simulink model "Dnote3lv3rd"  (R2016b)
settings: Solver=FixedStepDiscrete  StartTime=0.0  StopTime=simtime  RelTol=1e-3  EnableMultiTasking=on
PreLoadFcn:
  | simtime=0.0034;
undefined symbols (not defined in the file): Amp, fdesignblkfcn, Fin, Fs, FSC, gcbh, N, p, sw1, Ts
libraries: simulink x153, dspsnks4 x2, dspfdesign x1, dspvision x1, dsparch4 x1, dspmlti4 x1
(part 2 of 3)

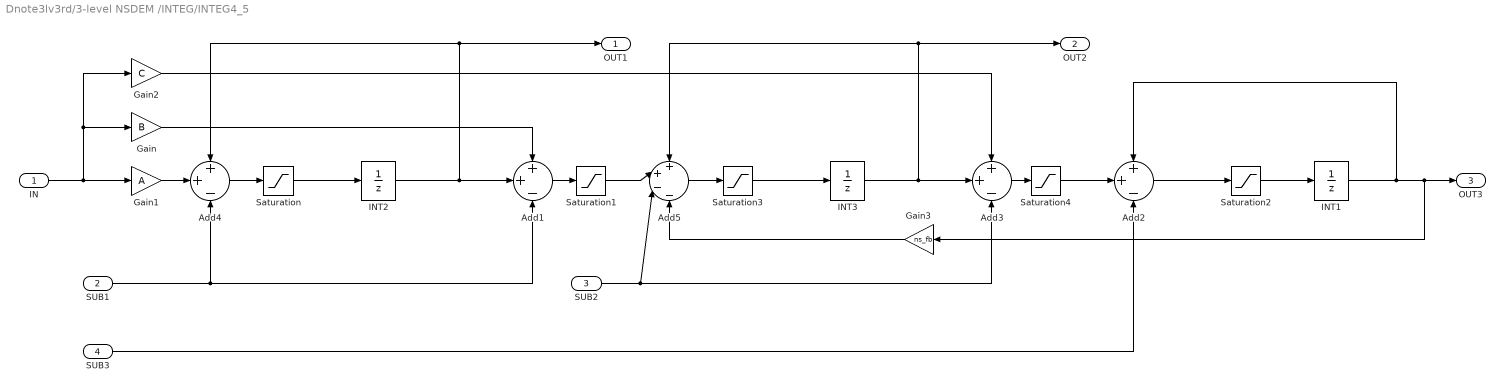
== system Dnote3lv3rd/3-level NSDEM /INTEG/INTEG4_5 ==
  IN : Inport
  SUB1 : Inport  Port=2
  SUB2 : Inport  Port=3
  SUB3 : Inport  Port=4
  Add{1..4} (4 alike) : Sum  Inputs=++-
  Add5 : Sum  Inputs=++--
  Gain : Gain  Gain=B
  Gain1 : Gain  Gain=A
  Gain2 : Gain  Gain=C
  Gain3 : Gain  Gain=ns_fb
  INT1 : UnitDelay  SampleTime=Ts
  INT2 : UnitDelay  SampleTime=Ts
  INT3 : UnitDelay  SampleTime=Ts
  Saturation{,1..4} (5 alike) : Saturate  UpperLimit=SAT  LowerLimit=-SAT
  OUT1 : Outport
  OUT2 : Outport  Port=2
  OUT3 : Outport  Port=3
  wires:
  Gain1/1 -> Add4/2
  Saturation1/1 -> Add5/2
  Saturation4/1 -> Add2/2
  Gain2/1 -> Add3/1
  Add3/1 -> Saturation4/1
  SUB2/1 -> Add3/3, Add5/3
  Add5/1 -> Saturation3/1
  Add2/1 -> Saturation2/1
  Gain/1 -> Add1/1
  Add1/1 -> Saturation1/1
  IN/1 -> Gain1/1, Gain2/1, Gain/1
  SUB1/1 -> Add4/3, Add1/3
  Add4/1 -> Saturation/1
  SUB3/1 -> Add2/3
  Gain3/1 -> Add5/4
  INT1/1 -> Add2/1, Gain3/1, OUT3/1
  INT3/1 -> Add3/2, OUT2/1, Add5/1
  Saturation2/1 -> INT1/1
  INT2/1 -> OUT1/1, Add4/1, Add1/2
  Saturation/1 -> INT2/1
  Saturation3/1 -> INT3/1

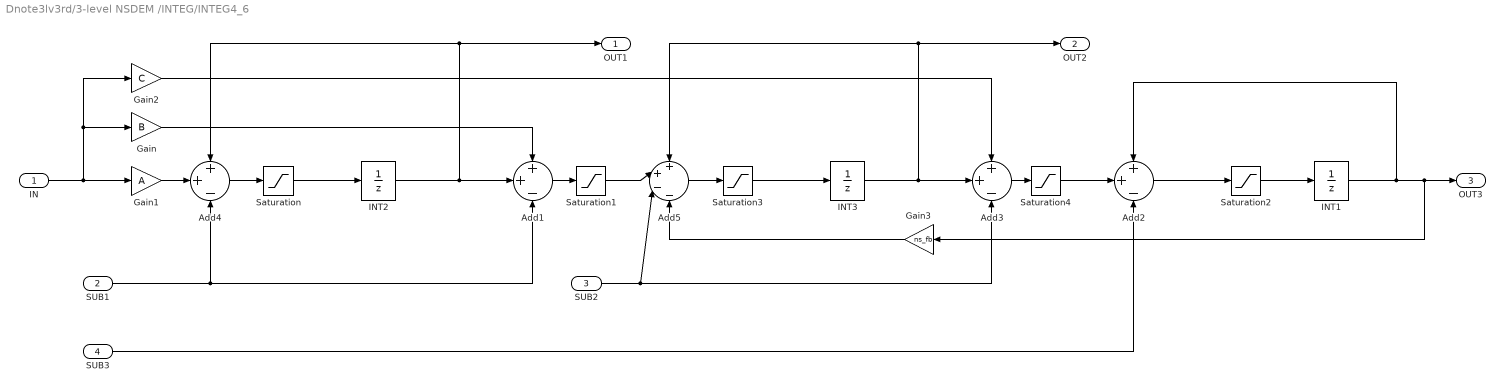
== system Dnote3lv3rd/3-level NSDEM /INTEG/INTEG4_6 ==
  IN : Inport
  SUB1 : Inport  Port=2
  SUB2 : Inport  Port=3
  SUB3 : Inport  Port=4
  Add{1..4} (4 alike) : Sum  Inputs=++-
  Add5 : Sum  Inputs=++--
  Gain : Gain  Gain=B
  Gain1 : Gain  Gain=A
  Gain2 : Gain  Gain=C
  Gain3 : Gain  Gain=ns_fb
  INT1 : UnitDelay  SampleTime=Ts
  INT2 : UnitDelay  SampleTime=Ts
  INT3 : UnitDelay  SampleTime=Ts
  Saturation{,1..4} (5 alike) : Saturate  UpperLimit=SAT  LowerLimit=-SAT
  OUT1 : Outport
  OUT2 : Outport  Port=2
  OUT3 : Outport  Port=3
  wires:
  Gain1/1 -> Add4/2
  Saturation1/1 -> Add5/2
  Saturation4/1 -> Add2/2
  Gain2/1 -> Add3/1
  Add3/1 -> Saturation4/1
  SUB2/1 -> Add3/3, Add5/3
  Add5/1 -> Saturation3/1
  Add2/1 -> Saturation2/1
  Gain/1 -> Add1/1
  Add1/1 -> Saturation1/1
  IN/1 -> Gain1/1, Gain2/1, Gain/1
  SUB1/1 -> Add4/3, Add1/3
  Add4/1 -> Saturation/1
  SUB3/1 -> Add2/3
  Gain3/1 -> Add5/4
  INT1/1 -> Add2/1, Gain3/1, OUT3/1
  INT3/1 -> Add3/2, OUT2/1, Add5/1
  Saturation2/1 -> INT1/1
  INT2/1 -> OUT1/1, Add4/1, Add1/2
  Saturation/1 -> INT2/1
  Saturation3/1 -> INT3/1

== system Dnote3lv3rd/3-level NSDEM /INTEG/INTEG4_7 ==
  IN : Inport
  SUB1 : Inport  Port=2
  SUB2 : Inport  Port=3
  SUB3 : Inport  Port=4
  Add{1..4} (4 alike) : Sum  Inputs=++-
  Add5 : Sum  Inputs=++--
  Gain : Gain  Gain=B
  Gain1 : Gain  Gain=A
  Gain2 : Gain  Gain=C
  Gain3 : Gain  Gain=ns_fb
  INT1 : UnitDelay  SampleTime=Ts
  INT2 : UnitDelay  SampleTime=Ts
  INT3 : UnitDelay  SampleTime=Ts
  Saturation{,1..4} (5 alike) : Saturate  UpperLimit=SAT  LowerLimit=-SAT
  OUT1 : Outport
  OUT2 : Outport  Port=2
  OUT3 : Outport  Port=3
  wires:
  Gain1/1 -> Add4/2
  Saturation1/1 -> Add5/2
  Saturation4/1 -> Add2/2
  Gain2/1 -> Add3/1
  Add3/1 -> Saturation4/1
  SUB2/1 -> Add3/3, Add5/3
  Add5/1 -> Saturation3/1
  Add2/1 -> Saturation2/1
  Gain/1 -> Add1/1
  Add1/1 -> Saturation1/1
  IN/1 -> Gain1/1, Gain2/1, Gain/1
  SUB1/1 -> Add4/3, Add1/3
  Add4/1 -> Saturation/1
  SUB3/1 -> Add2/3
  Gain3/1 -> Add5/4
  INT1/1 -> Add2/1, Gain3/1, OUT3/1
  INT3/1 -> Add3/2, OUT2/1, Add5/1
  Saturation2/1 -> INT1/1
  INT2/1 -> OUT1/1, Add4/1, Add1/2
  Saturation/1 -> INT2/1
  Saturation3/1 -> INT3/1

== system Dnote3lv3rd/3-level NSDEM /INTEG/INTEG4_8 ==
  IN : Inport
  SUB1 : Inport  Port=2
  SUB2 : Inport  Port=3
  SUB3 : Inport  Port=4
  Add{1..4} (4 alike) : Sum  Inputs=++-
  Add5 : Sum  Inputs=++--
  Gain : Gain  Gain=B
  Gain1 : Gain  Gain=A
  Gain2 : Gain  Gain=C
  Gain3 : Gain  Gain=ns_fb
  INT1 : UnitDelay  SampleTime=Ts
  INT2 : UnitDelay  SampleTime=Ts
  INT3 : UnitDelay  SampleTime=Ts
  Saturation{,1..4} (5 alike) : Saturate  UpperLimit=SAT  LowerLimit=-SAT
  OUT1 : Outport
  OUT2 : Outport  Port=2
  OUT3 : Outport  Port=3
  wires:
  Gain1/1 -> Add4/2
  Saturation1/1 -> Add5/2
  Saturation4/1 -> Add2/2
  Gain2/1 -> Add3/1
  Add3/1 -> Saturation4/1
  SUB2/1 -> Add3/3, Add5/3
  Add5/1 -> Saturation3/1
  Add2/1 -> Saturation2/1
  Gain/1 -> Add1/1
  Add1/1 -> Saturation1/1
  IN/1 -> Gain1/1, Gain2/1, Gain/1
  SUB1/1 -> Add4/3, Add1/3
  Add4/1 -> Saturation/1
  SUB3/1 -> Add2/3
  Gain3/1 -> Add5/4
  INT1/1 -> Add2/1, Gain3/1, OUT3/1
  INT3/1 -> Add3/2, OUT2/1, Add5/1
  Saturation2/1 -> INT1/1
  INT2/1 -> OUT1/1, Add4/1, Add1/2
  Saturation/1 -> INT2/1
  Saturation3/1 -> INT3/1

== system Dnote3lv3rd/3-level NSDEM /N_SELECTOR/Subsystem ==
  In1 : Inport
  Combinatorial Logic : CombinatorialLogic  TruthTable=[0 0 0 0 0 0 0 0;1 0 0 0 0 0 0 0]
  Combinatorial Logic1 : CombinatorialLogic  TruthTable=[0 0 0 0 0 0 0 0; 0 1 0 0 0 0 0 0]
  Combinatorial Logic2 : CombinatorialLogic  TruthTable=[0 0 0 0 0 0 0 0;0 0 1 0 0 0 0 0]
  Combinatorial Logic3 : CombinatorialLogic  TruthTable=[0 0 0 0 0 0 0 0;0 0 0 1 0 0 0 0]
  Combinatorial Logic4 : CombinatorialLogic  TruthTable=[0 0 0 0 0 0 0 0;0 0 0 0 1 0 0 0]
  Combinatorial Logic5 : CombinatorialLogic  TruthTable=[0 0 0 0 0 0 0 0;0 0 0 0 0 1 0 0]
  Combinatorial Logic6 : CombinatorialLogic  TruthTable=[0 0 0 0 0 0 0 0;0 0 0 0 0 0 1 0]
  Combinatorial Logic7 : CombinatorialLogic  TruthTable=[0 0 0 0 0 0 0 0;0 0 0 0 0 0 0 1]
  Compare To Constnt : simulink/Logic and Bit Operations/Compare To Constant  relop===  const=0  OutDataTypeStr=boolean  ZeroCross=off
  Compare To Constnt1 : simulink/Logic and Bit Operations/Compare To Constant  relop===  const=1  OutDataTypeStr=boolean  ZeroCross=off
  Compare To Constnt2 : simulink/Logic and Bit Operations/Compare To Constant  relop===  const=2  OutDataTypeStr=boolean  ZeroCross=off
  Compare To Constnt3 : simulink/Logic and Bit Operations/Compare To Constant  relop===  const=3  OutDataTypeStr=boolean  ZeroCross=off
  Compare To Constnt4 : simulink/Logic and Bit Operations/Compare To Constant  relop===  const=4  OutDataTypeStr=boolean  ZeroCross=off
  Compare To Constnt5 : simulink/Logic and Bit Operations/Compare To Constant  relop===  const=5  OutDataTypeStr=boolean  ZeroCross=off
  Compare To Constnt6 : simulink/Logic and Bit Operations/Compare To Constant  relop===  const=6  OutDataTypeStr=boolean  ZeroCross=off
  Compare To Constnt7 : simulink/Logic and Bit Operations/Compare To Constant  relop===  const=7  OutDataTypeStr=boolean  ZeroCross=off
  Logical Operator : Logic  Operator=OR  Inputs=8  AllPortsSameDT=off  OutDataTypeStr=boolean
  Out1 : Outport
  wires:
  Logical Operator/1 -> Out1/1
  In1/1 -> Compare To Constnt5/1, Compare To Constnt6/1, Compare To Constnt7/1, Compare To Constnt4/1, Compare To Constnt3/1, Compare To Constnt2/1, Compare To Constnt1/1, Compare To Constnt/1
  Compare To Constnt/1 -> Combinatorial Logic/1
  Compare To Constnt1/1 -> Combinatorial Logic1/1
  Compare To Constnt2/1 -> Combinatorial Logic2/1
  Compare To Constnt3/1 -> Combinatorial Logic3/1
  Compare To Constnt4/1 -> Combinatorial Logic4/1
  Compare To Constnt5/1 -> Combinatorial Logic5/1
  Compare To Constnt6/1 -> Combinatorial Logic6/1
  Compare To Constnt7/1 -> Combinatorial Logic7/1
  Combinatorial Logic/1 -> Logical Operator/1
  Combinatorial Logic1/1 -> Logical Operator/2
  Combinatorial Logic2/1 -> Logical Operator/3
  Combinatorial Logic3/1 -> Logical Operator/4
  Combinatorial Logic4/1 -> Logical Operator/5
  Combinatorial Logic5/1 -> Logical Operator/6
  Combinatorial Logic6/1 -> Logical Operator/7
  Combinatorial Logic7/1 -> Logical Operator/8

== system Dnote3lv3rd/3-level NSDEM /N_SELECTOR/Subsystem1 ==
  In1 : Inport
  Combinatorial Logic : CombinatorialLogic  TruthTable=[0 0 0 0 0 0 0 0;1 0 0 0 0 0 0 0]
  Combinatorial Logic1 : CombinatorialLogic  TruthTable=[0 0 0 0 0 0 0 0; 0 1 0 0 0 0 0 0]
  Combinatorial Logic2 : CombinatorialLogic  TruthTable=[0 0 0 0 0 0 0 0;0 0 1 0 0 0 0 0]
  Combinatorial Logic3 : CombinatorialLogic  TruthTable=[0 0 0 0 0 0 0 0;0 0 0 1 0 0 0 0]
  Combinatorial Logic4 : CombinatorialLogic  TruthTable=[0 0 0 0 0 0 0 0;0 0 0 0 1 0 0 0]
  Combinatorial Logic5 : CombinatorialLogic  TruthTable=[0 0 0 0 0 0 0 0;0 0 0 0 0 1 0 0]
  Combinatorial Logic6 : CombinatorialLogic  TruthTable=[0 0 0 0 0 0 0 0;0 0 0 0 0 0 1 0]
  Combinatorial Logic7 : CombinatorialLogic  TruthTable=[0 0 0 0 0 0 0 0;0 0 0 0 0 0 0 1]
  Compare To Constnt : simulink/Logic and Bit Operations/Compare To Constant  relop===  const=0  OutDataTypeStr=boolean  ZeroCross=off
  Compare To Constnt1 : simulink/Logic and Bit Operations/Compare To Constant  relop===  const=1  OutDataTypeStr=boolean  ZeroCross=off
  Compare To Constnt2 : simulink/Logic and Bit Operations/Compare To Constant  relop===  const=2  OutDataTypeStr=boolean  ZeroCross=off
  Compare To Constnt3 : simulink/Logic and Bit Operations/Compare To Constant  relop===  const=3  OutDataTypeStr=boolean  ZeroCross=off
  Compare To Constnt4 : simulink/Logic and Bit Operations/Compare To Constant  relop===  const=4  OutDataTypeStr=boolean  ZeroCross=off
  Compare To Constnt5 : simulink/Logic and Bit Operations/Compare To Constant  relop===  const=5  OutDataTypeStr=boolean  ZeroCross=off
  Compare To Constnt6 : simulink/Logic and Bit Operations/Compare To Constant  relop===  const=6  OutDataTypeStr=boolean  ZeroCross=off
  Compare To Constnt7 : simulink/Logic and Bit Operations/Compare To Constant  relop===  const=7  OutDataTypeStr=boolean  ZeroCross=off
  Logical Operator : Logic  Operator=OR  Inputs=8  AllPortsSameDT=off  OutDataTypeStr=boolean
  Out1 : Outport
  wires:
  Logical Operator/1 -> Out1/1
  In1/1 -> Compare To Constnt5/1, Compare To Constnt6/1, Compare To Constnt7/1, Compare To Constnt4/1, Compare To Constnt3/1, Compare To Constnt2/1, Compare To Constnt1/1, Compare To Constnt/1
  Compare To Constnt/1 -> Combinatorial Logic/1
  Compare To Constnt1/1 -> Combinatorial Logic1/1
  Compare To Constnt2/1 -> Combinatorial Logic2/1
  Compare To Constnt3/1 -> Combinatorial Logic3/1
  Compare To Constnt4/1 -> Combinatorial Logic4/1
  Compare To Constnt5/1 -> Combinatorial Logic5/1
  Compare To Constnt6/1 -> Combinatorial Logic6/1
  Compare To Constnt7/1 -> Combinatorial Logic7/1
  Combinatorial Logic/1 -> Logical Operator/1
  Combinatorial Logic1/1 -> Logical Operator/2
  Combinatorial Logic2/1 -> Logical Operator/3
  Combinatorial Logic3/1 -> Logical Operator/4
  Combinatorial Logic4/1 -> Logical Operator/5
  Combinatorial Logic5/1 -> Logical Operator/6
  Combinatorial Logic6/1 -> Logical Operator/7
  Combinatorial Logic7/1 -> Logical Operator/8

== system Dnote3lv3rd/3-level NSDEM /N_SELECTOR/Subsystem2 ==
  In1 : Inport
  Combinatorial Logic : CombinatorialLogic  TruthTable=[0 0 0 0 0 0 0 0;1 0 0 0 0 0 0 0]
  Combinatorial Logic1 : CombinatorialLogic  TruthTable=[0 0 0 0 0 0 0 0; 0 1 0 0 0 0 0 0]
  Combinatorial Logic2 : CombinatorialLogic  TruthTable=[0 0 0 0 0 0 0 0;0 0 1 0 0 0 0 0]
  Combinatorial Logic3 : CombinatorialLogic  TruthTable=[0 0 0 0 0 0 0 0;0 0 0 1 0 0 0 0]
  Combinatorial Logic4 : CombinatorialLogic  TruthTable=[0 0 0 0 0 0 0 0;0 0 0 0 1 0 0 0]
  Combinatorial Logic5 : CombinatorialLogic  TruthTable=[0 0 0 0 0 0 0 0;0 0 0 0 0 1 0 0]
  Combinatorial Logic6 : CombinatorialLogic  TruthTable=[0 0 0 0 0 0 0 0;0 0 0 0 0 0 1 0]
  Combinatorial Logic7 : CombinatorialLogic  TruthTable=[0 0 0 0 0 0 0 0;0 0 0 0 0 0 0 1]
  Compare To Constnt : simulink/Logic and Bit Operations/Compare To Constant  relop===  const=0  OutDataTypeStr=boolean  ZeroCross=off
  Compare To Constnt1 : simulink/Logic and Bit Operations/Compare To Constant  relop===  const=1  OutDataTypeStr=boolean  ZeroCross=off
  Compare To Constnt2 : simulink/Logic and Bit Operations/Compare To Constant  relop===  const=2  OutDataTypeStr=boolean  ZeroCross=off
  Compare To Constnt3 : simulink/Logic and Bit Operations/Compare To Constant  relop===  const=3  OutDataTypeStr=boolean  ZeroCross=off
  Compare To Constnt4 : simulink/Logic and Bit Operations/Compare To Constant  relop===  const=4  OutDataTypeStr=boolean  ZeroCross=off
  Compare To Constnt5 : simulink/Logic and Bit Operations/Compare To Constant  relop===  const=5  OutDataTypeStr=boolean  ZeroCross=off
  Compare To Constnt6 : simulink/Logic and Bit Operations/Compare To Constant  relop===  const=6  OutDataTypeStr=boolean  ZeroCross=off
  Compare To Constnt7 : simulink/Logic and Bit Operations/Compare To Constant  relop===  const=7  OutDataTypeStr=boolean  ZeroCross=off
  Logical Operator : Logic  Operator=OR  Inputs=8  AllPortsSameDT=off  OutDataTypeStr=boolean
  Out1 : Outport
  wires:
  Logical Operator/1 -> Out1/1
  In1/1 -> Compare To Constnt5/1, Compare To Constnt6/1, Compare To Constnt7/1, Compare To Constnt4/1, Compare To Constnt3/1, Compare To Constnt2/1, Compare To Constnt1/1, Compare To Constnt/1
  Compare To Constnt/1 -> Combinatorial Logic/1
  Compare To Constnt1/1 -> Combinatorial Logic1/1
  Compare To Constnt2/1 -> Combinatorial Logic2/1
  Compare To Constnt3/1 -> Combinatorial Logic3/1
  Compare To Constnt4/1 -> Combinatorial Logic4/1
  Compare To Constnt5/1 -> Combinatorial Logic5/1
  Compare To Constnt6/1 -> Combinatorial Logic6/1
  Compare To Constnt7/1 -> Combinatorial Logic7/1
  Combinatorial Logic/1 -> Logical Operator/1
  Combinatorial Logic1/1 -> Logical Operator/2
  Combinatorial Logic2/1 -> Logical Operator/3
  Combinatorial Logic3/1 -> Logical Operator/4
  Combinatorial Logic4/1 -> Logical Operator/5
  Combinatorial Logic5/1 -> Logical Operator/6
  Combinatorial Logic6/1 -> Logical Operator/7
  Combinatorial Logic7/1 -> Logical Operator/8

== system Dnote3lv3rd/3-level NSDEM /N_SELECTOR/Subsystem3 ==
  In1 : Inport
  Combinatorial Logic : CombinatorialLogic  TruthTable=[0 0 0 0 0 0 0 0;1 0 0 0 0 0 0 0]
  Combinatorial Logic1 : CombinatorialLogic  TruthTable=[0 0 0 0 0 0 0 0; 0 1 0 0 0 0 0 0]
  Combinatorial Logic2 : CombinatorialLogic  TruthTable=[0 0 0 0 0 0 0 0;0 0 1 0 0 0 0 0]
  Combinatorial Logic3 : CombinatorialLogic  TruthTable=[0 0 0 0 0 0 0 0;0 0 0 1 0 0 0 0]
  Combinatorial Logic4 : CombinatorialLogic  TruthTable=[0 0 0 0 0 0 0 0;0 0 0 0 1 0 0 0]
  Combinatorial Logic5 : CombinatorialLogic  TruthTable=[0 0 0 0 0 0 0 0;0 0 0 0 0 1 0 0]
  Combinatorial Logic6 : CombinatorialLogic  TruthTable=[0 0 0 0 0 0 0 0;0 0 0 0 0 0 1 0]
  Combinatorial Logic7 : CombinatorialLogic  TruthTable=[0 0 0 0 0 0 0 0;0 0 0 0 0 0 0 1]
  Compare To Constnt : simulink/Logic and Bit Operations/Compare To Constant  relop===  const=0  OutDataTypeStr=boolean  ZeroCross=off
  Compare To Constnt1 : simulink/Logic and Bit Operations/Compare To Constant  relop===  const=1  OutDataTypeStr=boolean  ZeroCross=off
  Compare To Constnt2 : simulink/Logic and Bit Operations/Compare To Constant  relop===  const=2  OutDataTypeStr=boolean  ZeroCross=off
  Compare To Constnt3 : simulink/Logic and Bit Operations/Compare To Constant  relop===  const=3  OutDataTypeStr=boolean  ZeroCross=off
  Compare To Constnt4 : simulink/Logic and Bit Operations/Compare To Constant  relop===  const=4  OutDataTypeStr=boolean  ZeroCross=off
  Compare To Constnt5 : simulink/Logic and Bit Operations/Compare To Constant  relop===  const=5  OutDataTypeStr=boolean  ZeroCross=off
  Compare To Constnt6 : simulink/Logic and Bit Operations/Compare To Constant  relop===  const=6  OutDataTypeStr=boolean  ZeroCross=off
  Compare To Constnt7 : simulink/Logic and Bit Operations/Compare To Constant  relop===  const=7  OutDataTypeStr=boolean  ZeroCross=off
  Logical Operator : Logic  Operator=OR  Inputs=8  AllPortsSameDT=off  OutDataTypeStr=boolean
  Out1 : Outport
  wires:
  Logical Operator/1 -> Out1/1
  In1/1 -> Compare To Constnt5/1, Compare To Constnt6/1, Compare To Constnt7/1, Compare To Constnt4/1, Compare To Constnt3/1, Compare To Constnt2/1, Compare To Constnt1/1, Compare To Constnt/1
  Compare To Constnt/1 -> Combinatorial Logic/1
  Compare To Constnt1/1 -> Combinatorial Logic1/1
  Compare To Constnt2/1 -> Combinatorial Logic2/1
  Compare To Constnt3/1 -> Combinatorial Logic3/1
  Compare To Constnt4/1 -> Combinatorial Logic4/1
  Compare To Constnt5/1 -> Combinatorial Logic5/1
  Compare To Constnt6/1 -> Combinatorial Logic6/1
  Compare To Constnt7/1 -> Combinatorial Logic7/1
  Combinatorial Logic/1 -> Logical Operator/1
  Combinatorial Logic1/1 -> Logical Operator/2
  Combinatorial Logic2/1 -> Logical Operator/3
  Combinatorial Logic3/1 -> Logical Operator/4
  Combinatorial Logic4/1 -> Logical Operator/5
  Combinatorial Logic5/1 -> Logical Operator/6
  Combinatorial Logic6/1 -> Logical Operator/7
  Combinatorial Logic7/1 -> Logical Operator/8

== system Dnote3lv3rd/3-level NSDEM /N_SELECTOR/Subsystem4 ==
  In1 : Inport
  Combinatorial Logic : CombinatorialLogic  TruthTable=[0 0 0 0 0 0 0 0;1 0 0 0 0 0 0 0]
  Combinatorial Logic1 : CombinatorialLogic  TruthTable=[0 0 0 0 0 0 0 0; 0 1 0 0 0 0 0 0]
  Combinatorial Logic2 : CombinatorialLogic  TruthTable=[0 0 0 0 0 0 0 0;0 0 1 0 0 0 0 0]
  Combinatorial Logic3 : CombinatorialLogic  TruthTable=[0 0 0 0 0 0 0 0;0 0 0 1 0 0 0 0]
  Combinatorial Logic4 : CombinatorialLogic  TruthTable=[0 0 0 0 0 0 0 0;0 0 0 0 1 0 0 0]
  Combinatorial Logic5 : CombinatorialLogic  TruthTable=[0 0 0 0 0 0 0 0;0 0 0 0 0 1 0 0]
  Combinatorial Logic6 : CombinatorialLogic  TruthTable=[0 0 0 0 0 0 0 0;0 0 0 0 0 0 1 0]
  Combinatorial Logic7 : CombinatorialLogic  TruthTable=[0 0 0 0 0 0 0 0;0 0 0 0 0 0 0 1]
  Compare To Constnt : simulink/Logic and Bit Operations/Compare To Constant  relop===  const=0  OutDataTypeStr=boolean  ZeroCross=off
  Compare To Constnt1 : simulink/Logic and Bit Operations/Compare To Constant  relop===  const=1  OutDataTypeStr=boolean  ZeroCross=off
  Compare To Constnt2 : simulink/Logic and Bit Operations/Compare To Constant  relop===  const=2  OutDataTypeStr=boolean  ZeroCross=off
  Compare To Constnt3 : simulink/Logic and Bit Operations/Compare To Constant  relop===  const=3  OutDataTypeStr=boolean  ZeroCross=off
  Compare To Constnt4 : simulink/Logic and Bit Operations/Compare To Constant  relop===  const=4  OutDataTypeStr=boolean  ZeroCross=off
  Compare To Constnt5 : simulink/Logic and Bit Operations/Compare To Constant  relop===  const=5  OutDataTypeStr=boolean  ZeroCross=off
  Compare To Constnt6 : simulink/Logic and Bit Operations/Compare To Constant  relop===  const=6  OutDataTypeStr=boolean  ZeroCross=off
  Compare To Constnt7 : simulink/Logic and Bit Operations/Compare To Constant  relop===  const=7  OutDataTypeStr=boolean  ZeroCross=off
  Logical Operator : Logic  Operator=OR  Inputs=8  AllPortsSameDT=off  OutDataTypeStr=boolean
  Out1 : Outport
  wires:
  Logical Operator/1 -> Out1/1
  In1/1 -> Compare To Constnt5/1, Compare To Constnt6/1, Compare To Constnt7/1, Compare To Constnt4/1, Compare To Constnt3/1, Compare To Constnt2/1, Compare To Constnt1/1, Compare To Constnt/1
  Compare To Constnt/1 -> Combinatorial Logic/1
  Compare To Constnt1/1 -> Combinatorial Logic1/1
  Compare To Constnt2/1 -> Combinatorial Logic2/1
  Compare To Constnt3/1 -> Combinatorial Logic3/1
  Compare To Constnt4/1 -> Combinatorial Logic4/1
  Compare To Constnt5/1 -> Combinatorial Logic5/1
  Compare To Constnt6/1 -> Combinatorial Logic6/1
  Compare To Constnt7/1 -> Combinatorial Logic7/1
  Combinatorial Logic/1 -> Logical Operator/1
  Combinatorial Logic1/1 -> Logical Operator/2
  Combinatorial Logic2/1 -> Logical Operator/3
  Combinatorial Logic3/1 -> Logical Operator/4
  Combinatorial Logic4/1 -> Logical Operator/5
  Combinatorial Logic5/1 -> Logical Operator/6
  Combinatorial Logic6/1 -> Logical Operator/7
  Combinatorial Logic7/1 -> Logical Operator/8

== system Dnote3lv3rd/3-level NSDEM /N_SELECTOR/Subsystem5 ==
  In1 : Inport
  Combinatorial Logic : CombinatorialLogic  TruthTable=[0 0 0 0 0 0 0 0;1 0 0 0 0 0 0 0]
  Combinatorial Logic1 : CombinatorialLogic  TruthTable=[0 0 0 0 0 0 0 0; 0 1 0 0 0 0 0 0]
  Combinatorial Logic2 : CombinatorialLogic  TruthTable=[0 0 0 0 0 0 0 0;0 0 1 0 0 0 0 0]
  Combinatorial Logic3 : CombinatorialLogic  TruthTable=[0 0 0 0 0 0 0 0;0 0 0 1 0 0 0 0]
  Combinatorial Logic4 : CombinatorialLogic  TruthTable=[0 0 0 0 0 0 0 0;0 0 0 0 1 0 0 0]
  Combinatorial Logic5 : CombinatorialLogic  TruthTable=[0 0 0 0 0 0 0 0;0 0 0 0 0 1 0 0]
  Combinatorial Logic6 : CombinatorialLogic  TruthTable=[0 0 0 0 0 0 0 0;0 0 0 0 0 0 1 0]
  Combinatorial Logic7 : CombinatorialLogic  TruthTable=[0 0 0 0 0 0 0 0;0 0 0 0 0 0 0 1]
  Compare To Constnt : simulink/Logic and Bit Operations/Compare To Constant  relop===  const=0  OutDataTypeStr=boolean  ZeroCross=off
  Compare To Constnt1 : simulink/Logic and Bit Operations/Compare To Constant  relop===  const=1  OutDataTypeStr=boolean  ZeroCross=off
  Compare To Constnt2 : simulink/Logic and Bit Operations/Compare To Constant  relop===  const=2  OutDataTypeStr=boolean  ZeroCross=off
  Compare To Constnt3 : simulink/Logic and Bit Operations/Compare To Constant  relop===  const=3  OutDataTypeStr=boolean  ZeroCross=off
  Compare To Constnt4 : simulink/Logic and Bit Operations/Compare To Constant  relop===  const=4  OutDataTypeStr=boolean  ZeroCross=off
  Compare To Constnt5 : simulink/Logic and Bit Operations/Compare To Constant  relop===  const=5  OutDataTypeStr=boolean  ZeroCross=off
  Compare To Constnt6 : simulink/Logic and Bit Operations/Compare To Constant  relop===  const=6  OutDataTypeStr=boolean  ZeroCross=off
  Compare To Constnt7 : simulink/Logic and Bit Operations/Compare To Constant  relop===  const=7  OutDataTypeStr=boolean  ZeroCross=off
  Logical Operator : Logic  Operator=OR  Inputs=8  AllPortsSameDT=off  OutDataTypeStr=boolean
  Out1 : Outport
  wires:
  Logical Operator/1 -> Out1/1
  In1/1 -> Compare To Constnt5/1, Compare To Constnt6/1, Compare To Constnt7/1, Compare To Constnt4/1, Compare To Constnt3/1, Compare To Constnt2/1, Compare To Constnt1/1, Compare To Constnt/1
  Compare To Constnt/1 -> Combinatorial Logic/1
  Compare To Constnt1/1 -> Combinatorial Logic1/1
  Compare To Constnt2/1 -> Combinatorial Logic2/1
  Compare To Constnt3/1 -> Combinatorial Logic3/1
  Compare To Constnt4/1 -> Combinatorial Logic4/1
  Compare To Constnt5/1 -> Combinatorial Logic5/1
  Compare To Constnt6/1 -> Combinatorial Logic6/1
  Compare To Constnt7/1 -> Combinatorial Logic7/1
  Combinatorial Logic/1 -> Logical Operator/1
  Combinatorial Logic1/1 -> Logical Operator/2
  Combinatorial Logic2/1 -> Logical Operator/3
  Combinatorial Logic3/1 -> Logical Operator/4
  Combinatorial Logic4/1 -> Logical Operator/5
  Combinatorial Logic5/1 -> Logical Operator/6
  Combinatorial Logic6/1 -> Logical Operator/7
  Combinatorial Logic7/1 -> Logical Operator/8

== system Dnote3lv3rd/3-level NSDEM /N_SELECTOR/Subsystem6 ==
  In1 : Inport
  Combinatorial Logic : CombinatorialLogic  TruthTable=[0 0 0 0 0 0 0 0;1 0 0 0 0 0 0 0]
  Combinatorial Logic1 : CombinatorialLogic  TruthTable=[0 0 0 0 0 0 0 0; 0 1 0 0 0 0 0 0]
  Combinatorial Logic2 : CombinatorialLogic  TruthTable=[0 0 0 0 0 0 0 0;0 0 1 0 0 0 0 0]
  Combinatorial Logic3 : CombinatorialLogic  TruthTable=[0 0 0 0 0 0 0 0;0 0 0 1 0 0 0 0]
  Combinatorial Logic4 : CombinatorialLogic  TruthTable=[0 0 0 0 0 0 0 0;0 0 0 0 1 0 0 0]
  Combinatorial Logic5 : CombinatorialLogic  TruthTable=[0 0 0 0 0 0 0 0;0 0 0 0 0 1 0 0]
  Combinatorial Logic6 : CombinatorialLogic  TruthTable=[0 0 0 0 0 0 0 0;0 0 0 0 0 0 1 0]
  Combinatorial Logic7 : CombinatorialLogic  TruthTable=[0 0 0 0 0 0 0 0;0 0 0 0 0 0 0 1]
  Compare To Constnt : simulink/Logic and Bit Operations/Compare To Constant  relop===  const=0  OutDataTypeStr=boolean  ZeroCross=off
  Compare To Constnt1 : simulink/Logic and Bit Operations/Compare To Constant  relop===  const=1  OutDataTypeStr=boolean  ZeroCross=off
  Compare To Constnt2 : simulink/Logic and Bit Operations/Compare To Constant  relop===  const=2  OutDataTypeStr=boolean  ZeroCross=off
  Compare To Constnt3 : simulink/Logic and Bit Operations/Compare To Constant  relop===  const=3  OutDataTypeStr=boolean  ZeroCross=off
  Compare To Constnt4 : simulink/Logic and Bit Operations/Compare To Constant  relop===  const=4  OutDataTypeStr=boolean  ZeroCross=off
  Compare To Constnt5 : simulink/Logic and Bit Operations/Compare To Constant  relop===  const=5  OutDataTypeStr=boolean  ZeroCross=off
  Compare To Constnt6 : simulink/Logic and Bit Operations/Compare To Constant  relop===  const=6  OutDataTypeStr=boolean  ZeroCross=off
  Compare To Constnt7 : simulink/Logic and Bit Operations/Compare To Constant  relop===  const=7  OutDataTypeStr=boolean  ZeroCross=off
  Logical Operator : Logic  Operator=OR  Inputs=8  AllPortsSameDT=off  OutDataTypeStr=boolean
  Out1 : Outport
  wires:
  Logical Operator/1 -> Out1/1
  In1/1 -> Compare To Constnt5/1, Compare To Constnt6/1, Compare To Constnt7/1, Compare To Constnt4/1, Compare To Constnt3/1, Compare To Constnt2/1, Compare To Constnt1/1, Compare To Constnt/1
  Compare To Constnt/1 -> Combinatorial Logic/1
  Compare To Constnt1/1 -> Combinatorial Logic1/1
  Compare To Constnt2/1 -> Combinatorial Logic2/1
  Compare To Constnt3/1 -> Combinatorial Logic3/1
  Compare To Constnt4/1 -> Combinatorial Logic4/1
  Compare To Constnt5/1 -> Combinatorial Logic5/1
  Compare To Constnt6/1 -> Combinatorial Logic6/1
  Compare To Constnt7/1 -> Combinatorial Logic7/1
  Combinatorial Logic/1 -> Logical Operator/1
  Combinatorial Logic1/1 -> Logical Operator/2
  Combinatorial Logic2/1 -> Logical Operator/3
  Combinatorial Logic3/1 -> Logical Operator/4
  Combinatorial Logic4/1 -> Logical Operator/5
  Combinatorial Logic5/1 -> Logical Operator/6
  Combinatorial Logic6/1 -> Logical Operator/7
  Combinatorial Logic7/1 -> Logical Operator/8

== system Dnote3lv3rd/3-level NSDEM /N_SELECTOR/Subsystem7 ==
  In1 : Inport
  Combinatorial Logic : CombinatorialLogic  TruthTable=[0 0 0 0 0 0 0 0;1 0 0 0 0 0 0 0]
  Combinatorial Logic1 : CombinatorialLogic  TruthTable=[0 0 0 0 0 0 0 0; 0 1 0 0 0 0 0 0]
  Combinatorial Logic2 : CombinatorialLogic  TruthTable=[0 0 0 0 0 0 0 0;0 0 1 0 0 0 0 0]
  Combinatorial Logic3 : CombinatorialLogic  TruthTable=[0 0 0 0 0 0 0 0;0 0 0 1 0 0 0 0]
  Combinatorial Logic4 : CombinatorialLogic  TruthTable=[0 0 0 0 0 0 0 0;0 0 0 0 1 0 0 0]
  Combinatorial Logic5 : CombinatorialLogic  TruthTable=[0 0 0 0 0 0 0 0;0 0 0 0 0 1 0 0]
  Combinatorial Logic6 : CombinatorialLogic  TruthTable=[0 0 0 0 0 0 0 0;0 0 0 0 0 0 1 0]
  Combinatorial Logic7 : CombinatorialLogic  TruthTable=[0 0 0 0 0 0 0 0;0 0 0 0 0 0 0 1]
  Compare To Constnt : simulink/Logic and Bit Operations/Compare To Constant  relop===  const=0  OutDataTypeStr=boolean  ZeroCross=off
  Compare To Constnt1 : simulink/Logic and Bit Operations/Compare To Constant  relop===  const=1  OutDataTypeStr=boolean  ZeroCross=off
  Compare To Constnt2 : simulink/Logic and Bit Operations/Compare To Constant  relop===  const=2  OutDataTypeStr=boolean  ZeroCross=off
  Compare To Constnt3 : simulink/Logic and Bit Operations/Compare To Constant  relop===  const=3  OutDataTypeStr=boolean  ZeroCross=off
  Compare To Constnt4 : simulink/Logic and Bit Operations/Compare To Constant  relop===  const=4  OutDataTypeStr=boolean  ZeroCross=off
  Compare To Constnt5 : simulink/Logic and Bit Operations/Compare To Constant  relop===  const=5  OutDataTypeStr=boolean  ZeroCross=off
  Compare To Constnt6 : simulink/Logic and Bit Operations/Compare To Constant  relop===  const=6  OutDataTypeStr=boolean  ZeroCross=off
  Compare To Constnt7 : simulink/Logic and Bit Operations/Compare To Constant  relop===  const=7  OutDataTypeStr=boolean  ZeroCross=off
  Logical Operator : Logic  Operator=OR  Inputs=8  AllPortsSameDT=off  OutDataTypeStr=boolean
  Out1 : Outport
  wires:
  Logical Operator/1 -> Out1/1
  In1/1 -> Compare To Constnt5/1, Compare To Constnt6/1, Compare To Constnt7/1, Compare To Constnt4/1, Compare To Constnt3/1, Compare To Constnt2/1, Compare To Constnt1/1, Compare To Constnt/1
  Compare To Constnt/1 -> Combinatorial Logic/1
  Compare To Constnt1/1 -> Combinatorial Logic1/1
  Compare To Constnt2/1 -> Combinatorial Logic2/1
  Compare To Constnt3/1 -> Combinatorial Logic3/1
  Compare To Constnt4/1 -> Combinatorial Logic4/1
  Compare To Constnt5/1 -> Combinatorial Logic5/1
  Compare To Constnt6/1 -> Combinatorial Logic6/1
  Compare To Constnt7/1 -> Combinatorial Logic7/1
  Combinatorial Logic/1 -> Logical Operator/1
  Combinatorial Logic1/1 -> Logical Operator/2
  Combinatorial Logic2/1 -> Logical Operator/3
  Combinatorial Logic3/1 -> Logical Operator/4
  Combinatorial Logic4/1 -> Logical Operator/5
  Combinatorial Logic5/1 -> Logical Operator/6
  Combinatorial Logic6/1 -> Logical Operator/7
  Combinatorial Logic7/1 -> Logical Operator/8

== system Dnote3lv3rd/3-level NSDEM /P_SELECTOR/Subsystem ==
  In1 : Inport
  Combinatorial Logic : CombinatorialLogic  TruthTable=[0 0 0 0 0 0 0 0;1 0 0 0 0 0 0 0]
  Combinatorial Logic1 : CombinatorialLogic  TruthTable=[0 0 0 0 0 0 0 0; 0 1 0 0 0 0 0 0]
  Combinatorial Logic2 : CombinatorialLogic  TruthTable=[0 0 0 0 0 0 0 0;0 0 1 0 0 0 0 0]
  Combinatorial Logic3 : CombinatorialLogic  TruthTable=[0 0 0 0 0 0 0 0;0 0 0 1 0 0 0 0]
  Combinatorial Logic4 : CombinatorialLogic  TruthTable=[0 0 0 0 0 0 0 0;0 0 0 0 1 0 0 0]
  Combinatorial Logic5 : CombinatorialLogic  TruthTable=[0 0 0 0 0 0 0 0;0 0 0 0 0 1 0 0]
  Combinatorial Logic6 : CombinatorialLogic  TruthTable=[0 0 0 0 0 0 0 0;0 0 0 0 0 0 1 0]
  Combinatorial Logic7 : CombinatorialLogic  TruthTable=[0 0 0 0 0 0 0 0;0 0 0 0 0 0 0 1]
  Compare To Constnt : simulink/Logic and Bit Operations/Compare To Constant  relop===  const=0  OutDataTypeStr=boolean  ZeroCross=off
  Compare To Constnt1 : simulink/Logic and Bit Operations/Compare To Constant  relop===  const=1  OutDataTypeStr=boolean  ZeroCross=off
  Compare To Constnt2 : simulink/Logic and Bit Operations/Compare To Constant  relop===  const=2  OutDataTypeStr=boolean  ZeroCross=off
  Compare To Constnt3 : simulink/Logic and Bit Operations/Compare To Constant  relop===  const=3  OutDataTypeStr=boolean  ZeroCross=off
  Compare To Constnt4 : simulink/Logic and Bit Operations/Compare To Constant  relop===  const=4  OutDataTypeStr=boolean  ZeroCross=off
  Compare To Constnt5 : simulink/Logic and Bit Operations/Compare To Constant  relop===  const=5  OutDataTypeStr=boolean  ZeroCross=off
  Compare To Constnt6 : simulink/Logic and Bit Operations/Compare To Constant  relop===  const=6  OutDataTypeStr=boolean  ZeroCross=off
  Compare To Constnt7 : simulink/Logic and Bit Operations/Compare To Constant  relop===  const=7  OutDataTypeStr=boolean  ZeroCross=off
  Logical Operator : Logic  Operator=OR  Inputs=8  AllPortsSameDT=off  OutDataTypeStr=boolean
  Out1 : Outport
  wires:
  Logical Operator/1 -> Out1/1
  In1/1 -> Compare To Constnt5/1, Compare To Constnt6/1, Compare To Constnt7/1, Compare To Constnt4/1, Compare To Constnt3/1, Compare To Constnt2/1, Compare To Constnt1/1, Compare To Constnt/1
  Compare To Constnt/1 -> Combinatorial Logic/1
  Compare To Constnt1/1 -> Combinatorial Logic1/1
  Compare To Constnt2/1 -> Combinatorial Logic2/1
  Compare To Constnt3/1 -> Combinatorial Logic3/1
  Compare To Constnt4/1 -> Combinatorial Logic4/1
  Compare To Constnt5/1 -> Combinatorial Logic5/1
  Compare To Constnt6/1 -> Combinatorial Logic6/1
  Compare To Constnt7/1 -> Combinatorial Logic7/1
  Combinatorial Logic/1 -> Logical Operator/1
  Combinatorial Logic1/1 -> Logical Operator/2
  Combinatorial Logic2/1 -> Logical Operator/3
  Combinatorial Logic3/1 -> Logical Operator/4
  Combinatorial Logic4/1 -> Logical Operator/5
  Combinatorial Logic5/1 -> Logical Operator/6
  Combinatorial Logic6/1 -> Logical Operator/7
  Combinatorial Logic7/1 -> Logical Operator/8

== system Dnote3lv3rd/3-level NSDEM /P_SELECTOR/Subsystem1 ==
  In1 : Inport
  Combinatorial Logic : CombinatorialLogic  TruthTable=[0 0 0 0 0 0 0 0;1 0 0 0 0 0 0 0]
  Combinatorial Logic1 : CombinatorialLogic  TruthTable=[0 0 0 0 0 0 0 0; 0 1 0 0 0 0 0 0]
  Combinatorial Logic2 : CombinatorialLogic  TruthTable=[0 0 0 0 0 0 0 0;0 0 1 0 0 0 0 0]
  Combinatorial Logic3 : CombinatorialLogic  TruthTable=[0 0 0 0 0 0 0 0;0 0 0 1 0 0 0 0]
  Combinatorial Logic4 : CombinatorialLogic  TruthTable=[0 0 0 0 0 0 0 0;0 0 0 0 1 0 0 0]
  Combinatorial Logic5 : CombinatorialLogic  TruthTable=[0 0 0 0 0 0 0 0;0 0 0 0 0 1 0 0]
  Combinatorial Logic6 : CombinatorialLogic  TruthTable=[0 0 0 0 0 0 0 0;0 0 0 0 0 0 1 0]
  Combinatorial Logic7 : CombinatorialLogic  TruthTable=[0 0 0 0 0 0 0 0;0 0 0 0 0 0 0 1]
  Compare To Constnt : simulink/Logic and Bit Operations/Compare To Constant  relop===  const=0  OutDataTypeStr=boolean  ZeroCross=off
  Compare To Constnt1 : simulink/Logic and Bit Operations/Compare To Constant  relop===  const=1  OutDataTypeStr=boolean  ZeroCross=off
  Compare To Constnt2 : simulink/Logic and Bit Operations/Compare To Constant  relop===  const=2  OutDataTypeStr=boolean  ZeroCross=off
  Compare To Constnt3 : simulink/Logic and Bit Operations/Compare To Constant  relop===  const=3  OutDataTypeStr=boolean  ZeroCross=off
  Compare To Constnt4 : simulink/Logic and Bit Operations/Compare To Constant  relop===  const=4  OutDataTypeStr=boolean  ZeroCross=off
  Compare To Constnt5 : simulink/Logic and Bit Operations/Compare To Constant  relop===  const=5  OutDataTypeStr=boolean  ZeroCross=off
  Compare To Constnt6 : simulink/Logic and Bit Operations/Compare To Constant  relop===  const=6  OutDataTypeStr=boolean  ZeroCross=off
  Compare To Constnt7 : simulink/Logic and Bit Operations/Compare To Constant  relop===  const=7  OutDataTypeStr=boolean  ZeroCross=off
  Logical Operator : Logic  Operator=OR  Inputs=8  AllPortsSameDT=off  OutDataTypeStr=boolean
  Out1 : Outport
  wires:
  Logical Operator/1 -> Out1/1
  In1/1 -> Compare To Constnt5/1, Compare To Constnt6/1, Compare To Constnt7/1, Compare To Constnt4/1, Compare To Constnt3/1, Compare To Constnt2/1, Compare To Constnt1/1, Compare To Constnt/1
  Compare To Constnt/1 -> Combinatorial Logic/1
  Compare To Constnt1/1 -> Combinatorial Logic1/1
  Compare To Constnt2/1 -> Combinatorial Logic2/1
  Compare To Constnt3/1 -> Combinatorial Logic3/1
  Compare To Constnt4/1 -> Combinatorial Logic4/1
  Compare To Constnt5/1 -> Combinatorial Logic5/1
  Compare To Constnt6/1 -> Combinatorial Logic6/1
  Compare To Constnt7/1 -> Combinatorial Logic7/1
  Combinatorial Logic/1 -> Logical Operator/1
  Combinatorial Logic1/1 -> Logical Operator/2
  Combinatorial Logic2/1 -> Logical Operator/3
  Combinatorial Logic3/1 -> Logical Operator/4
  Combinatorial Logic4/1 -> Logical Operator/5
  Combinatorial Logic5/1 -> Logical Operator/6
  Combinatorial Logic6/1 -> Logical Operator/7
  Combinatorial Logic7/1 -> Logical Operator/8

== system Dnote3lv3rd/3-level NSDEM /P_SELECTOR/Subsystem2 ==
  In1 : Inport
  Combinatorial Logic : CombinatorialLogic  TruthTable=[0 0 0 0 0 0 0 0;1 0 0 0 0 0 0 0]
  Combinatorial Logic1 : CombinatorialLogic  TruthTable=[0 0 0 0 0 0 0 0; 0 1 0 0 0 0 0 0]
  Combinatorial Logic2 : CombinatorialLogic  TruthTable=[0 0 0 0 0 0 0 0;0 0 1 0 0 0 0 0]
  Combinatorial Logic3 : CombinatorialLogic  TruthTable=[0 0 0 0 0 0 0 0;0 0 0 1 0 0 0 0]
  Combinatorial Logic4 : CombinatorialLogic  TruthTable=[0 0 0 0 0 0 0 0;0 0 0 0 1 0 0 0]
  Combinatorial Logic5 : CombinatorialLogic  TruthTable=[0 0 0 0 0 0 0 0;0 0 0 0 0 1 0 0]
  Combinatorial Logic6 : CombinatorialLogic  TruthTable=[0 0 0 0 0 0 0 0;0 0 0 0 0 0 1 0]
  Combinatorial Logic7 : CombinatorialLogic  TruthTable=[0 0 0 0 0 0 0 0;0 0 0 0 0 0 0 1]
  Compare To Constnt : simulink/Logic and Bit Operations/Compare To Constant  relop===  const=0  OutDataTypeStr=boolean  ZeroCross=off
  Compare To Constnt1 : simulink/Logic and Bit Operations/Compare To Constant  relop===  const=1  OutDataTypeStr=boolean  ZeroCross=off
  Compare To Constnt2 : simulink/Logic and Bit Operations/Compare To Constant  relop===  const=2  OutDataTypeStr=boolean  ZeroCross=off
  Compare To Constnt3 : simulink/Logic and Bit Operations/Compare To Constant  relop===  const=3  OutDataTypeStr=boolean  ZeroCross=off
  Compare To Constnt4 : simulink/Logic and Bit Operations/Compare To Constant  relop===  const=4  OutDataTypeStr=boolean  ZeroCross=off
  Compare To Constnt5 : simulink/Logic and Bit Operations/Compare To Constant  relop===  const=5  OutDataTypeStr=boolean  ZeroCross=off
  Compare To Constnt6 : simulink/Logic and Bit Operations/Compare To Constant  relop===  const=6  OutDataTypeStr=boolean  ZeroCross=off
  Compare To Constnt7 : simulink/Logic and Bit Operations/Compare To Constant  relop===  const=7  OutDataTypeStr=boolean  ZeroCross=off
  Logical Operator : Logic  Operator=OR  Inputs=8  AllPortsSameDT=off  OutDataTypeStr=boolean
  Out1 : Outport
  wires:
  Logical Operator/1 -> Out1/1
  In1/1 -> Compare To Constnt5/1, Compare To Constnt6/1, Compare To Constnt7/1, Compare To Constnt4/1, Compare To Constnt3/1, Compare To Constnt2/1, Compare To Constnt1/1, Compare To Constnt/1
  Compare To Constnt/1 -> Combinatorial Logic/1
  Compare To Constnt1/1 -> Combinatorial Logic1/1
  Compare To Constnt2/1 -> Combinatorial Logic2/1
  Compare To Constnt3/1 -> Combinatorial Logic3/1
  Compare To Constnt4/1 -> Combinatorial Logic4/1
  Compare To Constnt5/1 -> Combinatorial Logic5/1
  Compare To Constnt6/1 -> Combinatorial Logic6/1
  Compare To Constnt7/1 -> Combinatorial Logic7/1
  Combinatorial Logic/1 -> Logical Operator/1
  Combinatorial Logic1/1 -> Logical Operator/2
  Combinatorial Logic2/1 -> Logical Operator/3
  Combinatorial Logic3/1 -> Logical Operator/4
  Combinatorial Logic4/1 -> Logical Operator/5
  Combinatorial Logic5/1 -> Logical Operator/6
  Combinatorial Logic6/1 -> Logical Operator/7
  Combinatorial Logic7/1 -> Logical Operator/8

== system Dnote3lv3rd/3-level NSDEM /P_SELECTOR/Subsystem3 ==
  In1 : Inport
  Combinatorial Logic : CombinatorialLogic  TruthTable=[0 0 0 0 0 0 0 0;1 0 0 0 0 0 0 0]
  Combinatorial Logic1 : CombinatorialLogic  TruthTable=[0 0 0 0 0 0 0 0; 0 1 0 0 0 0 0 0]
  Combinatorial Logic2 : CombinatorialLogic  TruthTable=[0 0 0 0 0 0 0 0;0 0 1 0 0 0 0 0]
  Combinatorial Logic3 : CombinatorialLogic  TruthTable=[0 0 0 0 0 0 0 0;0 0 0 1 0 0 0 0]
  Combinatorial Logic4 : CombinatorialLogic  TruthTable=[0 0 0 0 0 0 0 0;0 0 0 0 1 0 0 0]
  Combinatorial Logic5 : CombinatorialLogic  TruthTable=[0 0 0 0 0 0 0 0;0 0 0 0 0 1 0 0]
  Combinatorial Logic6 : CombinatorialLogic  TruthTable=[0 0 0 0 0 0 0 0;0 0 0 0 0 0 1 0]
  Combinatorial Logic7 : CombinatorialLogic  TruthTable=[0 0 0 0 0 0 0 0;0 0 0 0 0 0 0 1]
  Compare To Constnt : simulink/Logic and Bit Operations/Compare To Constant  relop===  const=0  OutDataTypeStr=boolean  ZeroCross=off
  Compare To Constnt1 : simulink/Logic and Bit Operations/Compare To Constant  relop===  const=1  OutDataTypeStr=boolean  ZeroCross=off
  Compare To Constnt2 : simulink/Logic and Bit Operations/Compare To Constant  relop===  const=2  OutDataTypeStr=boolean  ZeroCross=off
  Compare To Constnt3 : simulink/Logic and Bit Operations/Compare To Constant  relop===  const=3  OutDataTypeStr=boolean  ZeroCross=off
  Compare To Constnt4 : simulink/Logic and Bit Operations/Compare To Constant  relop===  const=4  OutDataTypeStr=boolean  ZeroCross=off
  Compare To Constnt5 : simulink/Logic and Bit Operations/Compare To Constant  relop===  const=5  OutDataTypeStr=boolean  ZeroCross=off
  Compare To Constnt6 : simulink/Logic and Bit Operations/Compare To Constant  relop===  const=6  OutDataTypeStr=boolean  ZeroCross=off
  Compare To Constnt7 : simulink/Logic and Bit Operations/Compare To Constant  relop===  const=7  OutDataTypeStr=boolean  ZeroCross=off
  Logical Operator : Logic  Operator=OR  Inputs=8  AllPortsSameDT=off  OutDataTypeStr=boolean
  Out1 : Outport
  wires:
  Logical Operator/1 -> Out1/1
  In1/1 -> Compare To Constnt5/1, Compare To Constnt6/1, Compare To Constnt7/1, Compare To Constnt4/1, Compare To Constnt3/1, Compare To Constnt2/1, Compare To Constnt1/1, Compare To Constnt/1
  Compare To Constnt/1 -> Combinatorial Logic/1
  Compare To Constnt1/1 -> Combinatorial Logic1/1
  Compare To Constnt2/1 -> Combinatorial Logic2/1
  Compare To Constnt3/1 -> Combinatorial Logic3/1
  Compare To Constnt4/1 -> Combinatorial Logic4/1
  Compare To Constnt5/1 -> Combinatorial Logic5/1
  Compare To Constnt6/1 -> Combinatorial Logic6/1
  Compare To Constnt7/1 -> Combinatorial Logic7/1
  Combinatorial Logic/1 -> Logical Operator/1
  Combinatorial Logic1/1 -> Logical Operator/2
  Combinatorial Logic2/1 -> Logical Operator/3
  Combinatorial Logic3/1 -> Logical Operator/4
  Combinatorial Logic4/1 -> Logical Operator/5
  Combinatorial Logic5/1 -> Logical Operator/6
  Combinatorial Logic6/1 -> Logical Operator/7
  Combinatorial Logic7/1 -> Logical Operator/8

== system Dnote3lv3rd/3-level NSDEM /P_SELECTOR/Subsystem4 ==
  In1 : Inport
  Combinatorial Logic : CombinatorialLogic  TruthTable=[0 0 0 0 0 0 0 0;1 0 0 0 0 0 0 0]
  Combinatorial Logic1 : CombinatorialLogic  TruthTable=[0 0 0 0 0 0 0 0; 0 1 0 0 0 0 0 0]
  Combinatorial Logic2 : CombinatorialLogic  TruthTable=[0 0 0 0 0 0 0 0;0 0 1 0 0 0 0 0]
  Combinatorial Logic3 : CombinatorialLogic  TruthTable=[0 0 0 0 0 0 0 0;0 0 0 1 0 0 0 0]
  Combinatorial Logic4 : CombinatorialLogic  TruthTable=[0 0 0 0 0 0 0 0;0 0 0 0 1 0 0 0]
  Combinatorial Logic5 : CombinatorialLogic  TruthTable=[0 0 0 0 0 0 0 0;0 0 0 0 0 1 0 0]
  Combinatorial Logic6 : CombinatorialLogic  TruthTable=[0 0 0 0 0 0 0 0;0 0 0 0 0 0 1 0]
  Combinatorial Logic7 : CombinatorialLogic  TruthTable=[0 0 0 0 0 0 0 0;0 0 0 0 0 0 0 1]
  Compare To Constnt : simulink/Logic and Bit Operations/Compare To Constant  relop===  const=0  OutDataTypeStr=boolean  ZeroCross=off
  Compare To Constnt1 : simulink/Logic and Bit Operations/Compare To Constant  relop===  const=1  OutDataTypeStr=boolean  ZeroCross=off
  Compare To Constnt2 : simulink/Logic and Bit Operations/Compare To Constant  relop===  const=2  OutDataTypeStr=boolean  ZeroCross=off
  Compare To Constnt3 : simulink/Logic and Bit Operations/Compare To Constant  relop===  const=3  OutDataTypeStr=boolean  ZeroCross=off
  Compare To Constnt4 : simulink/Logic and Bit Operations/Compare To Constant  relop===  const=4  OutDataTypeStr=boolean  ZeroCross=off
  Compare To Constnt5 : simulink/Logic and Bit Operations/Compare To Constant  relop===  const=5  OutDataTypeStr=boolean  ZeroCross=off
  Compare To Constnt6 : simulink/Logic and Bit Operations/Compare To Constant  relop===  const=6  OutDataTypeStr=boolean  ZeroCross=off
  Compare To Constnt7 : simulink/Logic and Bit Operations/Compare To Constant  relop===  const=7  OutDataTypeStr=boolean  ZeroCross=off
  Logical Operator : Logic  Operator=OR  Inputs=8  AllPortsSameDT=off  OutDataTypeStr=boolean
  Out1 : Outport
  wires:
  Logical Operator/1 -> Out1/1
  In1/1 -> Compare To Constnt5/1, Compare To Constnt6/1, Compare To Constnt7/1, Compare To Constnt4/1, Compare To Constnt3/1, Compare To Constnt2/1, Compare To Constnt1/1, Compare To Constnt/1
  Compare To Constnt/1 -> Combinatorial Logic/1
  Compare To Constnt1/1 -> Combinatorial Logic1/1
  Compare To Constnt2/1 -> Combinatorial Logic2/1
  Compare To Constnt3/1 -> Combinatorial Logic3/1
  Compare To Constnt4/1 -> Combinatorial Logic4/1
  Compare To Constnt5/1 -> Combinatorial Logic5/1
  Compare To Constnt6/1 -> Combinatorial Logic6/1
  Compare To Constnt7/1 -> Combinatorial Logic7/1
  Combinatorial Logic/1 -> Logical Operator/1
  Combinatorial Logic1/1 -> Logical Operator/2
  Combinatorial Logic2/1 -> Logical Operator/3
  Combinatorial Logic3/1 -> Logical Operator/4
  Combinatorial Logic4/1 -> Logical Operator/5
  Combinatorial Logic5/1 -> Logical Operator/6
  Combinatorial Logic6/1 -> Logical Operator/7
  Combinatorial Logic7/1 -> Logical Operator/8

== system Dnote3lv3rd/3-level NSDEM /P_SELECTOR/Subsystem5 ==
  In1 : Inport
  Combinatorial Logic : CombinatorialLogic  TruthTable=[0 0 0 0 0 0 0 0;1 0 0 0 0 0 0 0]
  Combinatorial Logic1 : CombinatorialLogic  TruthTable=[0 0 0 0 0 0 0 0; 0 1 0 0 0 0 0 0]
  Combinatorial Logic2 : CombinatorialLogic  TruthTable=[0 0 0 0 0 0 0 0;0 0 1 0 0 0 0 0]
  Combinatorial Logic3 : CombinatorialLogic  TruthTable=[0 0 0 0 0 0 0 0;0 0 0 1 0 0 0 0]
  Combinatorial Logic4 : CombinatorialLogic  TruthTable=[0 0 0 0 0 0 0 0;0 0 0 0 1 0 0 0]
  Combinatorial Logic5 : CombinatorialLogic  TruthTable=[0 0 0 0 0 0 0 0;0 0 0 0 0 1 0 0]
  Combinatorial Logic6 : CombinatorialLogic  TruthTable=[0 0 0 0 0 0 0 0;0 0 0 0 0 0 1 0]
  Combinatorial Logic7 : CombinatorialLogic  TruthTable=[0 0 0 0 0 0 0 0;0 0 0 0 0 0 0 1]
  Compare To Constnt : simulink/Logic and Bit Operations/Compare To Constant  relop===  const=0  OutDataTypeStr=boolean  ZeroCross=off
  Compare To Constnt1 : simulink/Logic and Bit Operations/Compare To Constant  relop===  const=1  OutDataTypeStr=boolean  ZeroCross=off
  Compare To Constnt2 : simulink/Logic and Bit Operations/Compare To Constant  relop===  const=2  OutDataTypeStr=boolean  ZeroCross=off
  Compare To Constnt3 : simulink/Logic and Bit Operations/Compare To Constant  relop===  const=3  OutDataTypeStr=boolean  ZeroCross=off
  Compare To Constnt4 : simulink/Logic and Bit Operations/Compare To Constant  relop===  const=4  OutDataTypeStr=boolean  ZeroCross=off
  Compare To Constnt5 : simulink/Logic and Bit Operations/Compare To Constant  relop===  const=5  OutDataTypeStr=boolean  ZeroCross=off
  Compare To Constnt6 : simulink/Logic and Bit Operations/Compare To Constant  relop===  const=6  OutDataTypeStr=boolean  ZeroCross=off
  Compare To Constnt7 : simulink/Logic and Bit Operations/Compare To Constant  relop===  const=7  OutDataTypeStr=boolean  ZeroCross=off
  Logical Operator : Logic  Operator=OR  Inputs=8  AllPortsSameDT=off  OutDataTypeStr=boolean
  Out1 : Outport
  wires:
  Logical Operator/1 -> Out1/1
  In1/1 -> Compare To Constnt5/1, Compare To Constnt6/1, Compare To Constnt7/1, Compare To Constnt4/1, Compare To Constnt3/1, Compare To Constnt2/1, Compare To Constnt1/1, Compare To Constnt/1
  Compare To Constnt/1 -> Combinatorial Logic/1
  Compare To Constnt1/1 -> Combinatorial Logic1/1
  Compare To Constnt2/1 -> Combinatorial Logic2/1
  Compare To Constnt3/1 -> Combinatorial Logic3/1
  Compare To Constnt4/1 -> Combinatorial Logic4/1
  Compare To Constnt5/1 -> Combinatorial Logic5/1
  Compare To Constnt6/1 -> Combinatorial Logic6/1
  Compare To Constnt7/1 -> Combinatorial Logic7/1
  Combinatorial Logic/1 -> Logical Operator/1
  Combinatorial Logic1/1 -> Logical Operator/2
  Combinatorial Logic2/1 -> Logical Operator/3
  Combinatorial Logic3/1 -> Logical Operator/4
  Combinatorial Logic4/1 -> Logical Operator/5
  Combinatorial Logic5/1 -> Logical Operator/6
  Combinatorial Logic6/1 -> Logical Operator/7
  Combinatorial Logic7/1 -> Logical Operator/8

== system Dnote3lv3rd/3-level NSDEM /P_SELECTOR/Subsystem6 ==
  In1 : Inport
  Combinatorial Logic : CombinatorialLogic  TruthTable=[0 0 0 0 0 0 0 0;1 0 0 0 0 0 0 0]
  Combinatorial Logic1 : CombinatorialLogic  TruthTable=[0 0 0 0 0 0 0 0; 0 1 0 0 0 0 0 0]
  Combinatorial Logic2 : CombinatorialLogic  TruthTable=[0 0 0 0 0 0 0 0;0 0 1 0 0 0 0 0]
  Combinatorial Logic3 : CombinatorialLogic  TruthTable=[0 0 0 0 0 0 0 0;0 0 0 1 0 0 0 0]
  Combinatorial Logic4 : CombinatorialLogic  TruthTable=[0 0 0 0 0 0 0 0;0 0 0 0 1 0 0 0]
  Combinatorial Logic5 : CombinatorialLogic  TruthTable=[0 0 0 0 0 0 0 0;0 0 0 0 0 1 0 0]
  Combinatorial Logic6 : CombinatorialLogic  TruthTable=[0 0 0 0 0 0 0 0;0 0 0 0 0 0 1 0]
  Combinatorial Logic7 : CombinatorialLogic  TruthTable=[0 0 0 0 0 0 0 0;0 0 0 0 0 0 0 1]
  Compare To Constnt : simulink/Logic and Bit Operations/Compare To Constant  relop===  const=0  OutDataTypeStr=boolean  ZeroCross=off
  Compare To Constnt1 : simulink/Logic and Bit Operations/Compare To Constant  relop===  const=1  OutDataTypeStr=boolean  ZeroCross=off
  Compare To Constnt2 : simulink/Logic and Bit Operations/Compare To Constant  relop===  const=2  OutDataTypeStr=boolean  ZeroCross=off
  Compare To Constnt3 : simulink/Logic and Bit Operations/Compare To Constant  relop===  const=3  OutDataTypeStr=boolean  ZeroCross=off
  Compare To Constnt4 : simulink/Logic and Bit Operations/Compare To Constant  relop===  const=4  OutDataTypeStr=boolean  ZeroCross=off
  Compare To Constnt5 : simulink/Logic and Bit Operations/Compare To Constant  relop===  const=5  OutDataTypeStr=boolean  ZeroCross=off
  Compare To Constnt6 : simulink/Logic and Bit Operations/Compare To Constant  relop===  const=6  OutDataTypeStr=boolean  ZeroCross=off
  Compare To Constnt7 : simulink/Logic and Bit Operations/Compare To Constant  relop===  const=7  OutDataTypeStr=boolean  ZeroCross=off
  Logical Operator : Logic  Operator=OR  Inputs=8  AllPortsSameDT=off  OutDataTypeStr=boolean
  Out1 : Outport
  wires:
  Logical Operator/1 -> Out1/1
  In1/1 -> Compare To Constnt5/1, Compare To Constnt6/1, Compare To Constnt7/1, Compare To Constnt4/1, Compare To Constnt3/1, Compare To Constnt2/1, Compare To Constnt1/1, Compare To Constnt/1
  Compare To Constnt/1 -> Combinatorial Logic/1
  Compare To Constnt1/1 -> Combinatorial Logic1/1
  Compare To Constnt2/1 -> Combinatorial Logic2/1
  Compare To Constnt3/1 -> Combinatorial Logic3/1
  Compare To Constnt4/1 -> Combinatorial Logic4/1
  Compare To Constnt5/1 -> Combinatorial Logic5/1
  Compare To Constnt6/1 -> Combinatorial Logic6/1
  Compare To Constnt7/1 -> Combinatorial Logic7/1
  Combinatorial Logic/1 -> Logical Operator/1
  Combinatorial Logic1/1 -> Logical Operator/2
  Combinatorial Logic2/1 -> Logical Operator/3
  Combinatorial Logic3/1 -> Logical Operator/4
  Combinatorial Logic4/1 -> Logical Operator/5
  Combinatorial Logic5/1 -> Logical Operator/6
  Combinatorial Logic6/1 -> Logical Operator/7
  Combinatorial Logic7/1 -> Logical Operator/8
